simulink model "QuickSyncDopplerLibrary"  (R2013a)
settings: Solver=ode3  StartTime=0  StopTime=1  FixedStep=2  RelTol=1e-3
undefined symbols (not defined in the file or in its folder): B, datafiI, datafiQ, i, magnitude, n, p, wholesignal
libraries: dspmtrx3 x8, UndergraduateResearch x6, dspxfrm3 x3, simulink x3, dspstat3 x2, dspindex x1
settings Model: Creator=dmiralles  LastModifiedBy=dmiralles

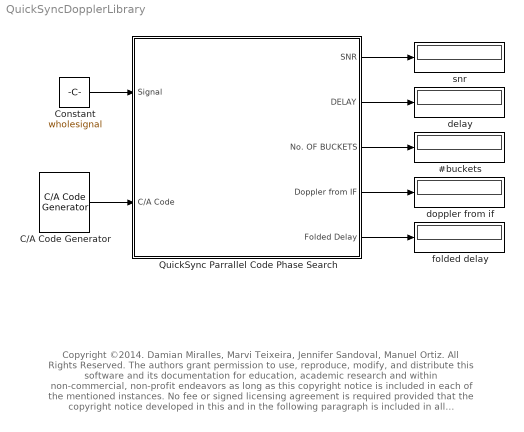
== system QuickSyncDopplerLibrary ==
  note: Copyright ©2014.  Damian Miralles, Marvi Teixeira, Jennifer Sandoval, Manuel Ortiz. All Rights Reserved.
      | The authors grant permission to use, reproduce, modify, and distribute this software and its documentation for
      | education,  academic research and within non-commercial, non-profit endeavors as long as this copyright notice
      |  is included in each of the mentioned instances. No fee or signed licensing agreement is required provided that
      | the copyright notice developed in this and in the following  paragraph is included in all reproductions,  alterations,
      | and distributions of the software or its  documentation. Contact the authors regarding any commercial licensing needs.
      |
      | THIS EXPERIMENTAL SOFTWARE AND RELATED DOCUMENTATION ARE PROVIDED “AS IS” AND
      |  NO, EXPLICIT OR IMPLICT, CLAIMS REGARDING THEIR ACCURACY OR SUITABILITY ARE MADE.
      | USERS ARE RESPONSIBLE FOR SOFTWARE VALIDATION REGARDING THEIR PARTICULAR
      |  APPLICATION. NO UPDATES WILL BE OFFERED. VERY LIMITED SUPPORT COULD BE PROVIDED,
      |  BUT NOT GUARANTEED, ON A CASE BY CASE BASIS, DEPENDING ON THE AVAILABLE TIME
      |  RESOURCES AT THE TIME OF THE REQUEST.
      | (dmiralles2009@gmail.com,  cc: mteixeir@ieee.org )
  " delay" : Display
  #buckets : Display
  C/A Code Generator : UndergraduateResearch/C//A Code Generator  fs=38192000  sat=22
  Constant : Constant  Value=wholesignal
  QuickSync Parrallel Code Phase Search : Subsystem  TreatAsAtomicUnit=on  mask{ssize=763840, ifreq=9548000, fs=38192000, satellite=21, threshold=22}
      mask prompts: ssize "Signal Size in Samples"; ifreq "Intermediate Frequency(Hz)"; fs "Sampling Frequency(Hz)"; satellite "Desired Satellite PRN"
      mask help:
      | The block implements the Parallel Code Search Acquisition method of a real time raw GPS signal. The block receives two input parameters, where signal is the raw gps signal and C/A code is the local generated code used as a method of comparison.
      | The block has several parameters to achieve its final functionality, the Signal Size is the size of the signal in samples that would be passed to the code, this value have to be an integer multiple of (sampling frequency/1000).
      | The intermediate frequency, expressed in Hertz , is the frequency to which the carrier frequency is shifted as an intermediate step in transmission or reception.
      | The sampling frequency defines the number of samples per unit of time (usually seconds) taken from a continuous signal to make a discrete signal.
      | The Desireed Satellite parameter defines the satellite that the user whcih to target in the simulation process if it is expected to be on the raw signal.
  doppler from if : Display
  folded delay : Display
  snr : Display
  wires:
  QuickSync Parrallel Code Phase Search/1(SNR) -> snr/1
  QuickSync Parrallel Code Phase Search/2(DELAY) -> " delay"/1
  QuickSync Parrallel Code Phase Search/3(No. OF BUCKETS) -> #buckets/1
  QuickSync Parrallel Code Phase Search/4(Doppler from IF) -> doppler from if/1
  Constant/1 -> QuickSync Parrallel Code Phase Search/1(Signal)
  C/A Code Generator/1 -> QuickSync Parrallel Code Phase Search/2(C/A Code)
  QuickSync Parrallel Code Phase Search/5(Folded Delay) -> folded delay/1

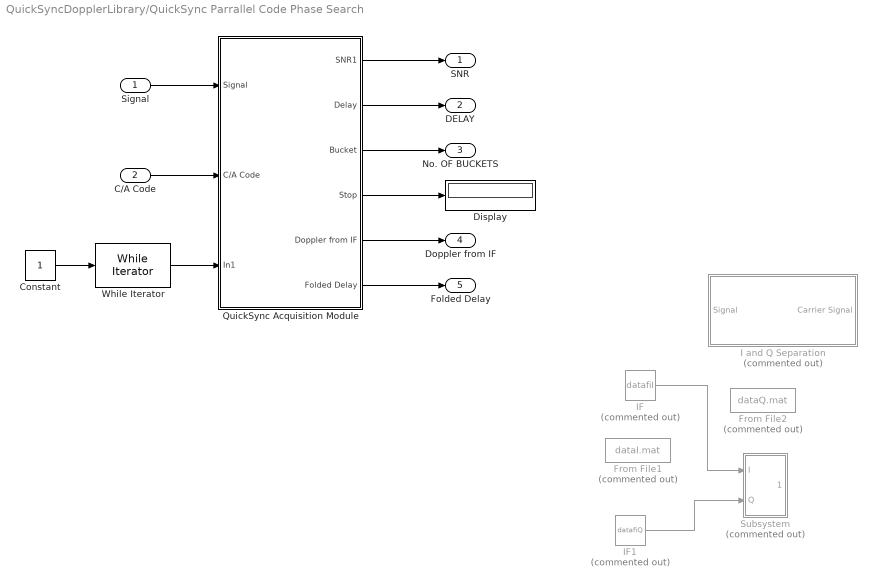
== system QuickSyncDopplerLibrary/QuickSync Parrallel Code Phase Search ==
  Signal : Inport
  C/A Code : Inport  Port=2
  Constant : Constant
  Display : Display
  From File1 : FromFile  Commented=on  FileName=dataI.mat  SampleTime=0
  From File2 : FromFile  Commented=on  FileName=dataQ.mat  SampleTime=0
  I and Q Separation : Subsystem  Commented=on  mask{ifreq=ifreq, ss=ssize, fs=fs}
      mask prompts: ifreq "Intermediate Frequency (Hz)"; ss "Signal Size"; fs "Sampling Frequency (Hz)"
  IF : Constant  Commented=on  Value=datafiI
  IF1 : Constant  Commented=on  Value=datafiQ
  QuickSync Acquisition Module : Subsystem  TreatAsAtomicUnit=on  mask{fs=fs}
      mask prompts: fs "Sampling Frequency"
  Subsystem : Subsystem  Commented=on
  While Iterator : WhileIterator  MaxIters=81  WhileBlockType=do-while  ResetStates=reset  ShowIterationPort=on  OutputDataType=int8
  SNR : Outport
  DELAY : Outport  Port=2
  No. OF BUCKETS : Outport  Port=3
  Doppler from IF : Outport  Port=4
  Folded Delay : Outport  Port=5
  wires:
  QuickSync Acquisition Module/1(SNR1) -> SNR/1
  QuickSync Acquisition Module/2(Delay) -> DELAY/1
  QuickSync Acquisition Module/3(Bucket) -> No. OF BUCKETS/1
  While Iterator/1 -> QuickSync Acquisition Module/3(In1)
  QuickSync Acquisition Module/5(Doppler from IF) -> Doppler from IF/1
  IF/1 -> Subsystem/1(I)
  IF1/1 -> Subsystem/2(Q)
  C/A Code/1 -> QuickSync Acquisition Module/2(C/A Code)
  Signal/1 -> QuickSync Acquisition Module/1(Signal)
  QuickSync Acquisition Module/6(Folded Delay) -> Folded Delay/1
  Constant/1 -> While Iterator/1
  QuickSync Acquisition Module/4(Stop) -> Display/1

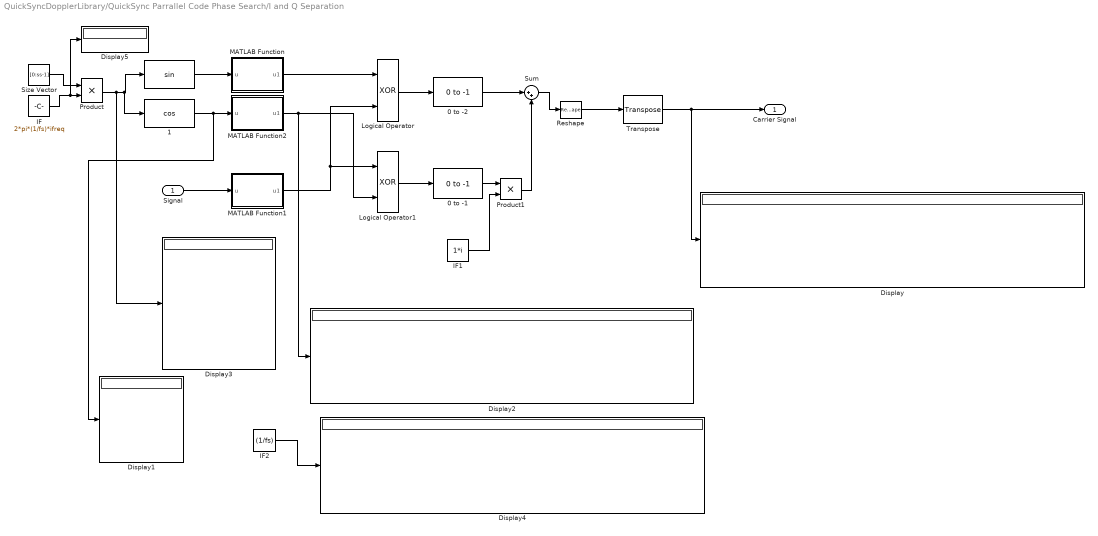
== system QuickSyncDopplerLibrary/QuickSync Parrallel Code Phase Search/I and Q Separation ==
  Signal : Inport
  " " : Trigonometry
  " 0 to -1" : UndergraduateResearch/ 0 to -1
  " 0 to -2" : UndergraduateResearch/ 0 to -1
  " 1" : Trigonometry  Operator=cos
  Display{,1..5} (6 alike) : Display
      Display4 settings: Format=long_e
  IF : Constant  Value=2*pi*(1/fs)*ifreq
  IF1 : Constant  Value=1*i
  IF2 : Constant  Value=(1/fs)
  Logical Operator : Logic  Operator=XOR  AllPortsSameDT=off  OutDataTypeStr=boolean
  Logical Operator1 : Logic  Operator=XOR  AllPortsSameDT=off  OutDataTypeStr=boolean
  MATLAB Function : MATLAB Function  TreatAsAtomicUnit=on
  MATLAB Function1 : MATLAB Function  TreatAsAtomicUnit=on
  MATLAB Function2 : MATLAB Function  TreatAsAtomicUnit=on
  Product : Product
  Product1 : Product
  Reshape : Reshape  OutputDimensionality=Customize  OutputDimensions=[38192,15]
  Size Vector : Constant  Value=[0:ss-1]
  Sum : Sum  Inputs=|++
  Transpose : dspmtrx3/Transpose  Hermitian=off  overflowFlag=off
  Carrier Signal : Outport
  wires:
  Size Vector/1 -> Product/1
  Product/1 -> Display3/1, " 1"/1, " "/1
  IF/1 -> Display5/1, Product/2
  Reshape/1 -> Transpose/1
  Transpose/1 -> Display/1, Carrier Signal/1
  " "/1 -> MATLAB Function/1(u)
  MATLAB Function/1(u1) -> Logical Operator/1
  MATLAB Function1/1(u1) -> Logical Operator1/1, Logical Operator/2
  Signal/1 -> MATLAB Function1/1(u)
  " 1"/1 -> Display1/1, MATLAB Function2/1(u)
  MATLAB Function2/1(u1) -> Display2/1, Logical Operator1/2
  Logical Operator1/1 -> " 0 to -1"/1
  Logical Operator/1 -> " 0 to -2"/1
  " 0 to -2"/1 -> Sum/1
  " 0 to -1"/1 -> Product1/1
  Product1/1 -> Sum/2
  IF1/1 -> Product1/2
  Sum/1 -> Reshape/1
  IF2/1 -> Display4/1

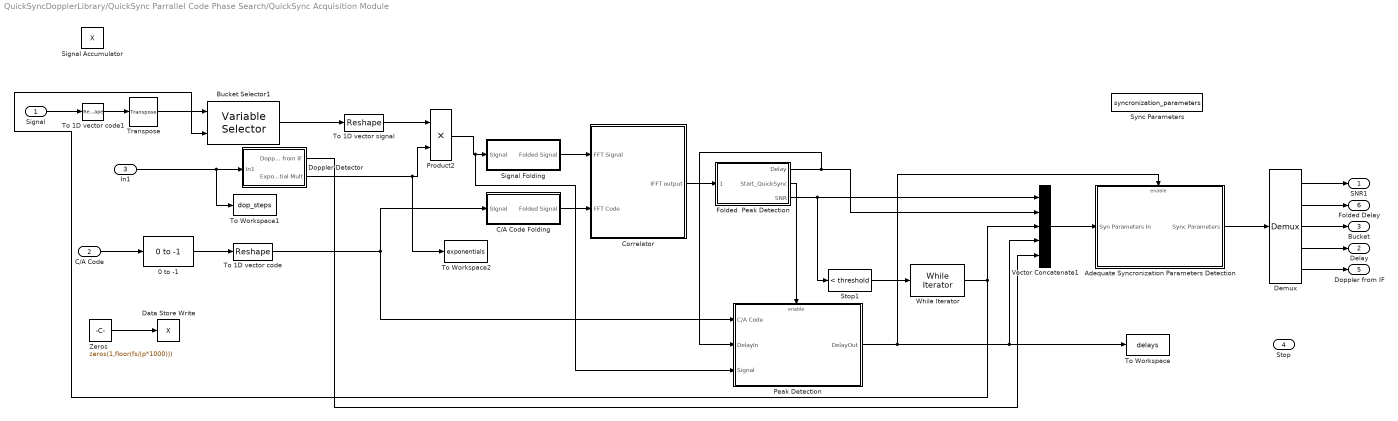
== system QuickSyncDopplerLibrary/QuickSync Parrallel Code Phase Search/QuickSync Acquisition Module ==
  Signal : Inport
  C/A Code : Inport  Port=2
  In1 : Inport  Port=3
  " 0 to -1" : UndergraduateResearch/ 0 to -1
  Adequate Syncronization Parameters Detection : Subsystem  TreatAsAtomicUnit=on
  Bucket Selector1 : dspindex/Variable Selector  NumInputs=1  rowsOrCols=Rows  IdxMode=Variable  Elements=[1 3]  ZerOneIdxMode=One-based  errmode=Clip Index  FillMode=on  FillValues=1
  C/A Code Folding : Subsystem
  Correlator : Subsystem
  Data Store Write : DataStoreWrite  DataStoreName=X
  Demux : Demux  Outputs=5
  Doppler Detector : Subsystem
  Folded  Peak Detection : Subsystem
      mask help: The Final block receives an IFFT and returns if the SNR passed the threshhold and also outputs the SNR and the delay. It uses a variable to accumulate the signal adds it to IFFT and stores it. It detects the maximum value in the signal with the index and assings a 0 to remove the peak to be able to calculate the mean and obtain the SNR.
  Peak Detection : Subsystem  TreatAsAtomicUnit=on
  Product2 : Product
  Signal Accumulator : DataStoreMemory  DataStoreName=X  ReadBeforeWriteMsg=warning  WriteAfterWriteMsg=warning  WriteAfterReadMsg=warning  InitialValue=zeros(1,floor(fs/(p*1000)))  VectorParams1D=off
  Signal Folding : Subsystem
  Stop1 : simulink/Logic and Bit Operations/Compare To Constant  relop=<  const=threshold  OutDataTypeStr=boolean
  Sync Parameters : DataStoreMemory  DataStoreName=syncronization_parameters  ReadBeforeWriteMsg=warning  WriteAfterWriteMsg=warning  WriteAfterReadMsg=warning  InitialValue=zeros(1,5)
  To 1D vector code : Reshape  OutputDimensions=[1023,40]
  To 1D vector code1 : Reshape  OutputDimensionality=Customize  OutputDimensions=[(n*p),ssize/(n*p)]
  To 1D vector signal : Reshape  OutputDimensions=[1023,40]
  To Workspace : ToWorkspace  VariableName=delays  SampleTime=-1
  To Workspace1 : ToWorkspace  VariableName=dop_steps  SampleTime=-1
  To Workspace2 : ToWorkspace  VariableName=exponentials  SampleTime=-1
  Transpose : dspmtrx3/Transpose  Hermitian=off  overflowFlag=off
  Vector Concatenate1 : Concatenate  NumInputs=5
  While Iterator : WhileIterator  WhileBlockType=do-while  ResetStates=reset  ShowIterationPort=on  OutputDataType=double
  Zeros : Constant  Value=zeros(1,floor(fs/(p*1000)))
  SNR1 : Outport
  Delay : Outport  Port=2
  Bucket : Outport  Port=3
  Stop : Outport  Port=4
  Doppler from IF : Outport  Port=5
  Folded Delay : Outport  Port=6
  wires:
  Folded  Peak Detection/3("SNR ") -> Vector Concatenate1/1, Stop1/1
  To 1D vector code/1 -> C/A Code Folding/1(SIgnal), Peak Detection/1("C/A Code ")
  C/A Code/1 -> " 0 to -1"/1
  " 0 to -1"/1 -> To 1D vector code/1
  Doppler Detector/1(Doppler from IF) -> Vector Concatenate1/5
  In1/1 -> To Workspace1/1, Doppler Detector/1(In1)
  Bucket Selector1/1 -> To 1D vector signal/1
  To 1D vector signal/1 -> Product2/1
  Zeros/1 -> Data Store Write/1
  Signal Folding/1(Folded Signal) -> Correlator/1(FFT Signal)
  C/A Code Folding/1(Folded Signal) -> Correlator/2(FFT Code)
  Product2/1 -> Peak Detection/3(Signal), Signal Folding/1(SIgnal)
  Correlator/1(IFFT output) -> Folded  Peak Detection/1("  ")
  Folded  Peak Detection/2(Start_QuickSync) -> Peak Detection/Enable
  Folded  Peak Detection/1(Delay) -> Vector Concatenate1/2, Peak Detection/2(DelayIn)
  Stop1/1 -> While Iterator/1
  Doppler Detector/2(Exponential Mult) -> To Workspace2/1, Product2/2
  While Iterator/1 -> Vector Concatenate1/3, Bucket Selector1/2
  To 1D vector code1/1 -> Transpose/1
  Signal/1 -> To 1D vector code1/1
  Transpose/1 -> Bucket Selector1/1
  Vector Concatenate1/1 -> Adequate Syncronization Parameters Detection/1(Syn Parameters In)
  Adequate Syncronization Parameters Detection/1("Sync Parameters ") -> Demux/1
  Demux/2 -> Folded Delay/1
  Demux/1 -> SNR1/1
  Demux/4 -> Delay/1
  Demux/3 -> Bucket/1
  Demux/5 -> Doppler from IF/1
  Peak Detection/1(DelayOut) -> Adequate Syncronization Parameters Detection/Enable, To Workspace/1, Vector Concatenate1/4

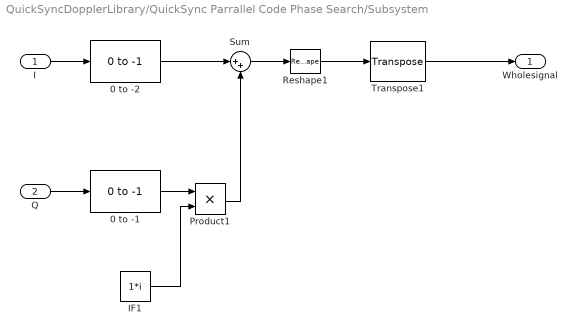
== system QuickSyncDopplerLibrary/QuickSync Parrallel Code Phase Search/Subsystem ==
  I : Inport
  Q : Inport  Port=2
  " 0 to -1" : UndergraduateResearch/ 0 to -1
  " 0 to -2" : UndergraduateResearch/ 0 to -1
  IF1 : Constant  Value=1*i
  Product1 : Product
  Reshape1 : Reshape  OutputDimensionality=Customize  OutputDimensions=[38192,15]
  Sum : Sum  Inputs=|++
  Transpose1 : dspmtrx3/Transpose  Hermitian=off  overflowFlag=off
  Wholesignal : Outport
  wires:
  " 0 to -2"/1 -> Sum/1
  Reshape1/1 -> Transpose1/1
  Transpose1/1 -> Wholesignal/1
  Sum/1 -> Reshape1/1
  Product1/1 -> Sum/2
  I/1 -> " 0 to -2"/1
  Q/1 -> " 0 to -1"/1
  " 0 to -1"/1 -> Product1/1
  IF1/1 -> Product1/2

== system QuickSyncDopplerLibrary/QuickSync Parrallel Code Phase Search/QuickSync Acquisition Module/Adequate Syncronization Parameters Detection ==
  Syn Parameters In : Inport
  Enable : EnablePort  StatesWhenEnabling=reset
  Demux : Demux  Outputs=5
  Read : DataStoreRead  DataStoreName=syncronization_parameters
  Relational Operator : RelationalOperator  OutDataTypeStr=boolean
  Switch : Switch  Criteria=u2 > Threshold
  Write : DataStoreWrite  DataStoreName=syncronization_parameters
  sync_par : ToWorkspace  VariableName=syn_parameters  SampleTime=-1
  "Sync Parameters " : Outport
  wires:
  Read/1 -> Switch/3, Relational Operator/2
  Switch/1 -> "Sync Parameters "/1, Write/1
  Syn Parameters In/1 -> Relational Operator/1, sync_par/1, Switch/1
  Relational Operator/1 -> Demux/1
  Demux/1 -> Switch/2

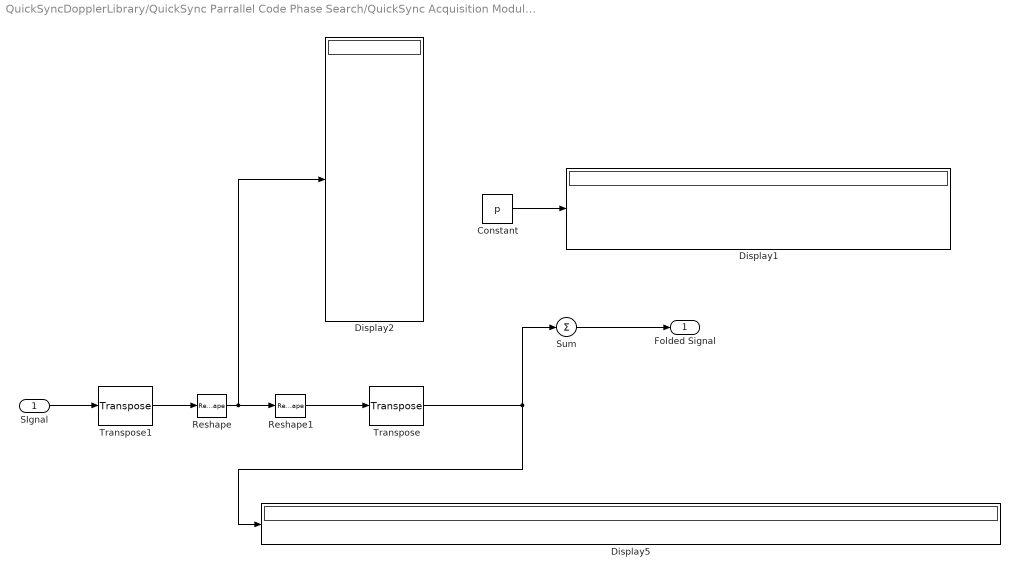
== system QuickSyncDopplerLibrary/QuickSync Parrallel Code Phase Search/QuickSync Acquisition Module/C//A Code Folding ==
  SIgnal : Inport
  Constant : Constant  Value=p
  Display1 : Display
  Display2 : Display
  Display5 : Display
  Reshape : Reshape
  Reshape1 : Reshape  OutputDimensionality=Customize  OutputDimensions=[(fs/1000)/p,p]
  Sum : Sum  Inputs=+  CollapseMode=Specified dimension
  Transpose : dspmtrx3/Transpose  Hermitian=off  overflowFlag=off
  Transpose1 : dspmtrx3/Transpose  Hermitian=off  overflowFlag=off
  Folded Signal : Outport
  wires:
  Transpose/1 -> Sum/1, Display5/1
  Sum/1 -> Folded Signal/1
  Reshape1/1 -> Transpose/1
  Constant/1 -> Display1/1
  SIgnal/1 -> Transpose1/1
  Transpose1/1 -> Reshape/1
  Reshape/1 -> Display2/1, Reshape1/1

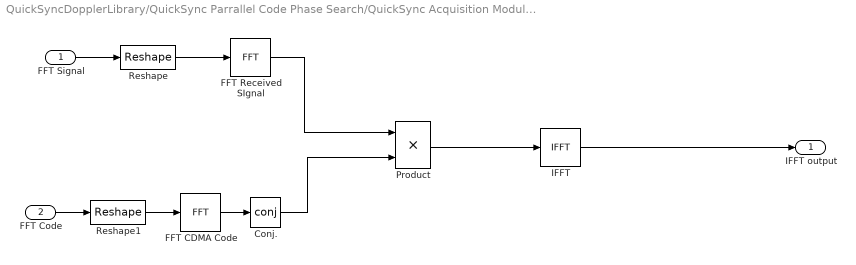
== system QuickSyncDopplerLibrary/QuickSync Parrallel Code Phase Search/QuickSync Acquisition Module/Correlator ==
  FFT Signal : Inport
  FFT Code : Inport  Port=2
  Conj. : Math  Operator=conj  SaturateOnIntegerOverflow=on
  FFT CDMA Code : dspxfrm3/FFT  CompMethod=Table lookup  TableOpt=NEW  TableOptActive=Speed  BitRevOrder=off  InheritFFTLength=on  FFTLength=1024  RowConvenienceOn=on  FFTImplementation=FFTW  SkipNorm=off  firstCoeffDataTypeStr=Inherit: Same word length as input  firstCoeffLastDataTypeStr=Inherit: Same word length as input  outputMin=[]  outputMax=[]  roundingMode=Floor  overflowMode=off
  FFT Received SIgnal : dspxfrm3/FFT  CompMethod=Table lookup  TableOpt=NEW  TableOptActive=Speed  BitRevOrder=off  InheritFFTLength=on  FFTLength=1024  RowConvenienceOn=on  FFTImplementation=FFTW  SkipNorm=off  firstCoeffDataTypeStr=Inherit: Same word length as input  firstCoeffLastDataTypeStr=Inherit: Same word length as input  outputMin=[]  outputMax=[]  roundingMode=Floor  overflowMode=off
  IFFT : dspxfrm3/IFFT  CompMethod=Table lookup  TableOpt=NEW  TableOptActive=Speed  BitRevOrder=off  cs_in=off  SkipNorm=on  InheritFFTLength=on  FFTLength=1024  mode=Complex  outSamplingMode=Sample based  RowConvenienceOn=on  FFTImplementation=FFTW  firstCoeffDataTypeStr=Inherit: Same word length as input  firstCoeffLastDataTypeStr=Inherit: Same word length as input  outputMin=[]  outputMax=[]  roundingMode=Floor  overflowMode=off
  Product : Product  RndMeth=Zero
  Reshape : Reshape  OutputDimensions=[1023,40]
  Reshape1 : Reshape  OutputDimensions=[1023,40]
  IFFT output : Outport
  wires:
  FFT Code/1 -> Reshape1/1
  Reshape1/1 -> FFT CDMA Code/1
  FFT Signal/1 -> Reshape/1
  Reshape/1 -> FFT Received SIgnal/1
  Product/1 -> IFFT/1
  Conj./1 -> Product/2
  FFT Received SIgnal/1 -> Product/1
  FFT CDMA Code/1 -> Conj./1
  IFFT/1 -> IFFT output/1

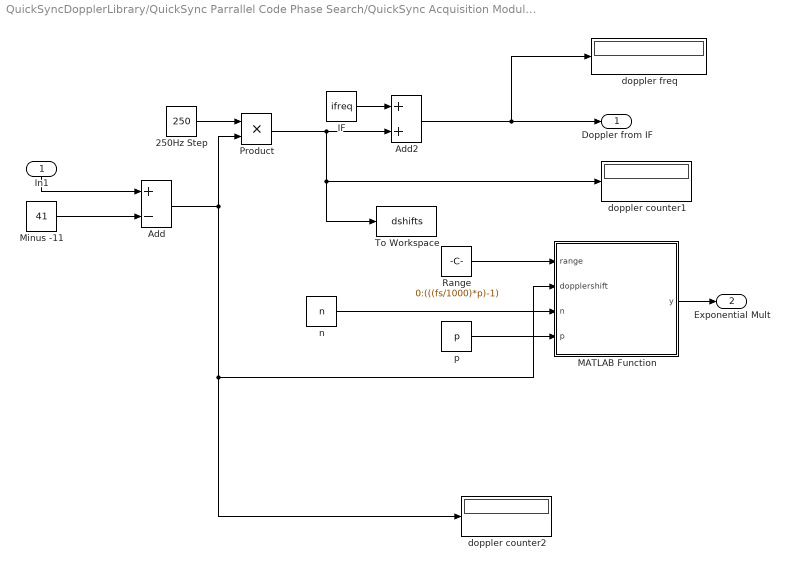
== system QuickSyncDopplerLibrary/QuickSync Parrallel Code Phase Search/QuickSync Acquisition Module/Doppler Detector ==
  In1 : Inport
  250Hz Step : Constant  Value=250
  Add : Sum  Inputs=+-
  Add2 : Sum
  IF : Constant  Value=ifreq
  MATLAB Function : MATLAB Function  TreatAsAtomicUnit=on
  Minus -11 : Constant  Value=41
  Product : Product
  Range : Constant  Value=0:(((fs/1000)*p)-1)
  To Workspace : ToWorkspace  VariableName=dshifts  SampleTime=-1
  doppler counter1 : Display
  doppler counter2 : Display
  doppler freq : Display
  n : Constant  Value=n
  p : Constant  Value=p
  Doppler from IF : Outport
  Exponential Mult : Outport  Port=2
  wires:
  Product/1 -> Add2/2, To Workspace/1, doppler counter1/1
  250Hz Step/1 -> Product/1
  Add2/1 -> doppler freq/1, Doppler from IF/1
  IF/1 -> Add2/1
  Minus -11/1 -> Add/2
  In1/1 -> Add/1
  Add/1 -> Product/2, MATLAB Function/2(dopplershift), doppler counter2/1
  Range/1 -> MATLAB Function/1(range)
  p/1 -> MATLAB Function/4(p)
  n/1 -> MATLAB Function/3(n)
  MATLAB Function/1(y) -> Exponential Mult/1

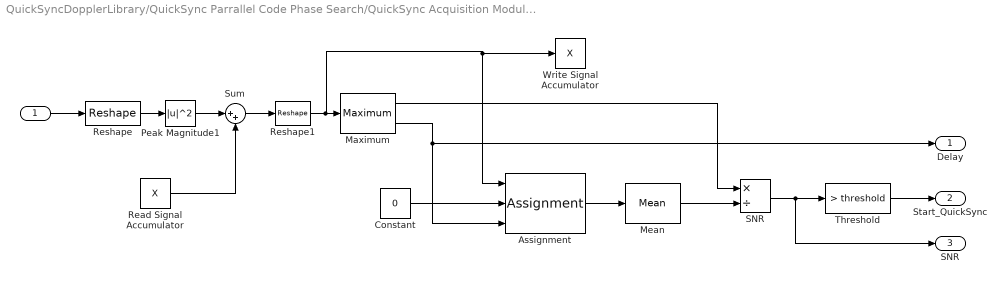
== system QuickSyncDopplerLibrary/QuickSync Parrallel Code Phase Search/QuickSync Acquisition Module/Folded  Peak Detection ==
  "  " : Inport
  " Read Signal Accumulator" : DataStoreRead  DataStoreName=X
  Assignment : Assignment  IndexOptions=Index vector (port)  Indices=1  OutputSizes=1
  Constant : Constant  Value=0
  Maximum : dspstat3/Maximum  fcn=Value and Index  reset=None  InputProcessing=Columns as channels (frame based)  indexBase=One  operateOver=Each column  Dimension=1  colComp=on  operation=maximum  roiEnable=off  roiType=Rectangles  roiPortion=Entire ROI  roiOutput=Individual statistics for each ROI  roiFlag=off  accumDataTypeStr=Inherit: Same as product output  accumLastDataTypeStr=Inherit: Same as product output  roundingMode=Floor  overflowMode=off
  Mean : dspstat3/Mean  run=off  reset_popup=None  InputProcessing=Columns as channels (frame based)  directionMode=Each column  dimension=1  treatSBRowAsCol=on  roiEnable=off  roiType=Rectangles  roiPortion=Entire ROI  roiOutput=Individual statistics for each ROI  roiFlag=off  outputDataTypeStr=Inherit: Same as accumulator  outputLastDataTypeStr=Inherit: Same as accumulator  outputMin=[]  outputMax=[]  roundingMode=Floor  overflowMode=off
  Peak Magnitude1 : Math  Operator=magnitude^2  SaturateOnIntegerOverflow=on
  Reshape : Reshape  OutputDimensions=[1023,40]
  Reshape1 : Reshape  OutputDimensions=[1023,40]
  SNR : Product  Inputs=*/
  Sum : Sum  Inputs=|++
  Threshold : simulink/Logic and Bit Operations/Compare To Constant  relop=>  const=threshold  OutDataTypeStr=boolean
  Write Signal Accumulator : DataStoreWrite  DataStoreName=X
  Delay : Outport
  Start_QuickSync : Outport  Port=2
  "SNR " : Outport  Port=3
  wires:
  "  "/1 -> Reshape/1
  Peak Magnitude1/1 -> Sum/1
  Constant/1 -> Assignment/2
  Assignment/1 -> Mean/1
  " Read Signal Accumulator"/1 -> Sum/2
  SNR/1 -> Threshold/1, "SNR "/1
  Mean/1 -> SNR/2
  Maximum/2 -> Assignment/3, Delay/1
  Threshold/1 -> Start_QuickSync/1
  Sum/1 -> Reshape1/1
  Maximum/1 -> SNR/1
  Reshape/1 -> Peak Magnitude1/1
  Reshape1/1 -> Maximum/1, Assignment/1, Write Signal Accumulator/1

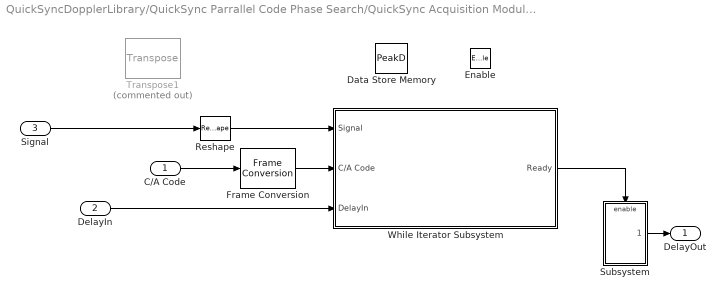
== system QuickSyncDopplerLibrary/QuickSync Parrallel Code Phase Search/QuickSync Acquisition Module/Peak Detection ==
  "C/A Code " : Inport
  DelayIn : Inport  Port=2
  Signal : Inport  Port=3
  Enable : EnablePort  StatesWhenEnabling=reset
  Data Store Memory : DataStoreMemory  DataStoreName=PeakD  ReadBeforeWriteMsg=warning  WriteAfterWriteMsg=warning  WriteAfterReadMsg=warning  InitialValue=zeros(1,2)  VectorParams1D=off
  Frame Conversion : FrameConversion  OutFrame=Sample-based
  Reshape : Reshape
  Subsystem : Subsystem
  Transpose1 : dspmtrx3/Transpose  Commented=on  Hermitian=off  overflowFlag=off
  While Iterator Subsystem : Subsystem  TreatAsAtomicUnit=on
  DelayOut : Outport
  wires:
  DelayIn/1 -> While Iterator Subsystem/3(DelayIn)
  While Iterator Subsystem/1(Ready) -> Subsystem/Enable
  Signal/1 -> Reshape/1
  Reshape/1 -> While Iterator Subsystem/1(Signal)
  "C/A Code "/1 -> Frame Conversion/1
  Frame Conversion/1 -> While Iterator Subsystem/2("C/A Code ")
  Subsystem/1(DelayOut) -> DelayOut/1

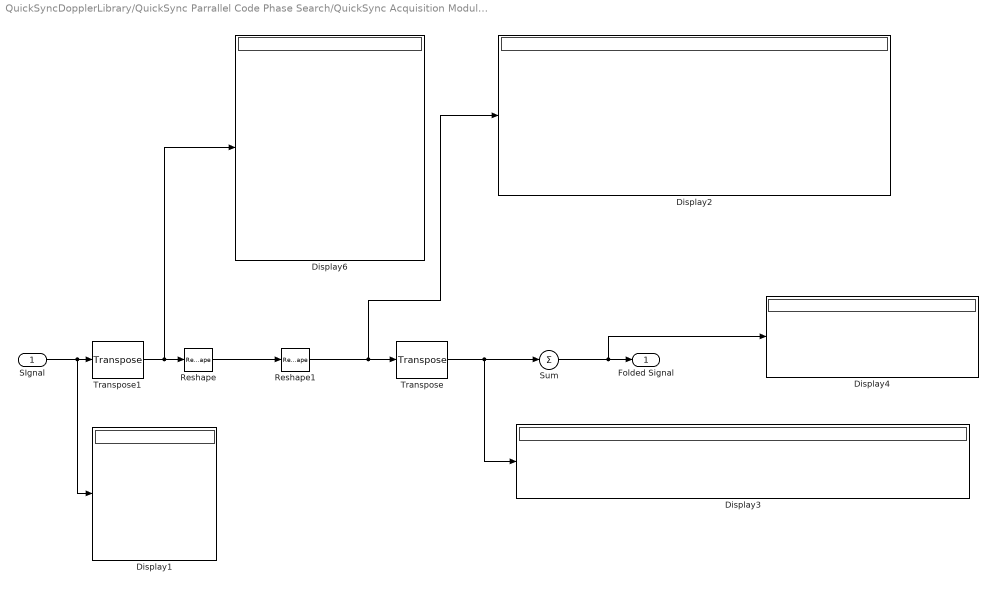
== system QuickSyncDopplerLibrary/QuickSync Parrallel Code Phase Search/QuickSync Acquisition Module/Signal Folding ==
  SIgnal : Inport
  Display{1..4,6} (5 alike) : Display
  Reshape : Reshape
  Reshape1 : Reshape  OutputDimensionality=Customize  OutputDimensions=[(fs/1000)/p,p^2]
  Sum : Sum  Inputs=+  CollapseMode=Specified dimension
  Transpose : dspmtrx3/Transpose  Hermitian=off  overflowFlag=off
  Transpose1 : dspmtrx3/Transpose  Hermitian=off  overflowFlag=off
  Folded Signal : Outport
  wires:
  Reshape/1 -> Reshape1/1
  Sum/1 -> Display4/1, Folded Signal/1
  SIgnal/1 -> Display1/1, Transpose1/1
  Transpose1/1 -> Display6/1, Reshape/1
  Reshape1/1 -> Display2/1, Transpose/1
  Transpose/1 -> Display3/1, Sum/1

== system QuickSyncDopplerLibrary/QuickSync Parrallel Code Phase Search/QuickSync Acquisition Module/Peak Detection/Subsystem ==
  Enable : EnablePort  StatesWhenEnabling=reset
  Data Store Read1 : DataStoreRead  DataStoreName=PeakD
  Demux : Demux  Outputs=2
  Value1 : Display
  DelayOut : Outport
  wires:
  Data Store Read1/1 -> Demux/1
  Demux/1 -> Value1/1
  Demux/2 -> DelayOut/1

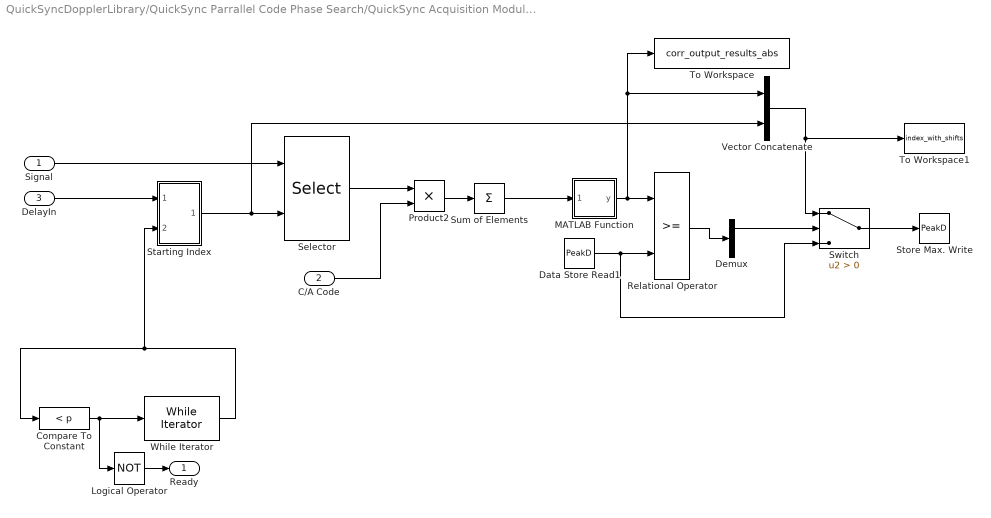
== system QuickSyncDopplerLibrary/QuickSync Parrallel Code Phase Search/QuickSync Acquisition Module/Peak Detection/While Iterator Subsystem ==
  Signal : Inport
  "C/A Code " : Inport  Port=2
  DelayIn : Inport  Port=3
  Compare To Constant : simulink/Logic and Bit Operations/Compare To Constant  relop=<  const=p  OutDataTypeStr=boolean
  Data Store Read1 : DataStoreRead  DataStoreName=PeakD
  Demux : Demux  Outputs=2
  Logical Operator : Logic  Operator=NOT  AllPortsSameDT=off  OutDataTypeStr=boolean
  MATLAB Function : MATLAB Function  TreatAsAtomicUnit=on
  Product2 : Product
  Relational Operator : RelationalOperator  OutDataTypeStr=boolean
  Selector : Selector  InputPortWidth=round(fs/1000)*p  IndexOptions=Starting index (port)  Indices=[1 3]  OutputSizes=round(fs/1000)
  Starting Index : Subsystem
  Store Max. Write : DataStoreWrite  DataStoreName=PeakD
  Sum of Elements : Sum  Inputs=+
  Switch : Switch  Criteria=u2 > Threshold
  To Workspace : ToWorkspace  VariableName=corr_output_results_abs  SampleTime=-1
  To Workspace1 : ToWorkspace  VariableName=index_with_shifts  SampleTime=-1
  Vector Concatenate : Concatenate
  While Iterator : WhileIterator  MaxIters=p  WhileBlockType=do-while  ResetStates=reset  ShowIterationPort=on
  Ready : Outport
  wires:
  "C/A Code "/1 -> Product2/2
  While Iterator/1 -> Starting Index/2(Counter), Compare To Constant/1
  Signal/1 -> Selector/1
  Starting Index/1(Index) -> Vector Concatenate/2, Selector/2
  Selector/1 -> Product2/1
  Product2/1 -> Sum of Elements/1
  Data Store Read1/1 -> Switch/3, Relational Operator/2
  Switch/1 -> Store Max. Write/1
  Compare To Constant/1 -> Logical Operator/1, While Iterator/1
  Logical Operator/1 -> Ready/1
  Vector Concatenate/1 -> To Workspace1/1, Switch/1
  DelayIn/1 -> Starting Index/1(DelayIn)
  Sum of Elements/1 -> MATLAB Function/1(signal)
  MATLAB Function/1(y) -> Relational Operator/1, Vector Concatenate/1, To Workspace/1
  Relational Operator/1 -> Demux/1
  Demux/1 -> Switch/2

== system QuickSyncDopplerLibrary/QuickSync Parrallel Code Phase Search/QuickSync Acquisition Module/Peak Detection/While Iterator Subsystem/Starting Index ==
  DelayIn : Inport
  Counter : Inport  Port=2
  B steps : Display
  Constant1 : Constant  Value=B
  Constant2 : Constant
  Product1 : Product
  Sum : Sum  Inputs=+-
  Sum1 : Sum  Inputs=|++
  Index : Outport
  wires:
  Counter/1 -> Sum/1
  Sum/1 -> Product1/1
  Constant2/1 -> Sum/2
  Constant1/1 -> Product1/2
  DelayIn/1 -> Sum1/1
  Product1/1 -> B steps/1, Sum1/2
  Sum1/1 -> Index/1

== matlab function QuickSyncDopplerLibrary/QuickSync Parrallel Code Phase Search/I and Q Separation/MATLAB Function1 ==
  data: u input; u1 output
function u1 = fcn(u)
%#codegen
u1 = u>0;

== matlab function QuickSyncDopplerLibrary/QuickSync Parrallel Code Phase Search/I and Q Separation/MATLAB Function ==
  data: u input; u1 output
function u1 = fcn(u)
%#codegen
u1 = u>0;

== matlab function QuickSyncDopplerLibrary/QuickSync Parrallel Code Phase Search/I and Q Separation/MATLAB Function2 ==
  data: u input; u1 output
function u1 = fcn(u)
%#codegen
u1=u>0;

== matlab function QuickSyncDopplerLibrary/QuickSync Parrallel Code Phase Search/QuickSync Acquisition Module/Doppler Detector/MATLAB Function ==
  data: range input; y output; dopplershift input; n input; p input
function y = exp(range,dopplershift,n,p)
%#codegen

y=exp(i*(2*pi/(n*p))*dopplershift.*range);

== matlab function QuickSyncDopplerLibrary/QuickSync Parrallel Code Phase Search/QuickSync Acquisition Module/Peak Detection/While Iterator Subsystem/MATLAB Function ==
  data: signal input; y output
function y = abs(signal)
%#codegen

y=abs(signal)
